simulink model "untitled"  (R2019b)
settings: Solver=VariableStepAuto  StartTime=0.0  StopTime=1.0  RelTol=1e-3
libraries: simulink x1
settings Model: Creator=patti  LastModifiedBy=patti

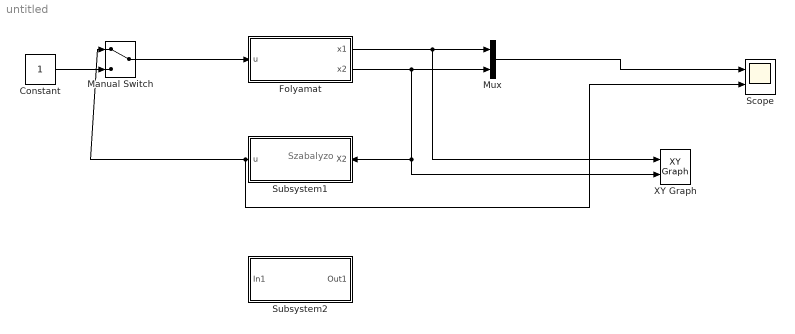
== system untitled ==
  note: Szabalyzo
  Constant : Constant
  "Folyamat " : Subsystem  mask{w=6, x0=[5  ; 8]}
  Manual Switch : ManualSwitch
  Mux : Mux  Inputs=2
  Scope : Scope  NumInputPorts=2
  Subsystem1 : Subsystem
  Subsystem2 : Subsystem
  XY Graph : simulink/Sinks/XY Graph  xmin=-10  xmax=100  ymin=-10  ymax=100  st=0.01
  wires:
  Manual Switch/1 -> "Folyamat "/1(u)
  "Folyamat "/1(x1) -> XY Graph/1, Mux/1
  "Folyamat "/2(x2) -> Mux/2, XY Graph/2, Subsystem1/1(X2)
  Subsystem1/1("u ") -> Scope/2, Manual Switch/1
  Constant/1 -> Manual Switch/2
  Mux/1 -> Scope/1

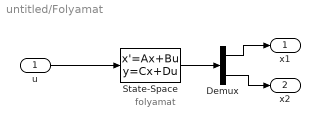
== system untitled/Folyamat  ==
  note: folyamat
  u : Inport
  Demux : Demux  Outputs=2
  State-Space : StateSpace  A=[0 w; -w 0]  B=[0 ; 1]  C=[1 0;0 1]  D=[0 ;0]  InitialCondition=[x0]
  x1 : Outport
  x2 : Outport  Port=2
  wires:
  u/1 -> State-Space/1
  State-Space/1 -> Demux/1
  Demux/1 -> x1/1
  Demux/2 -> x2/1

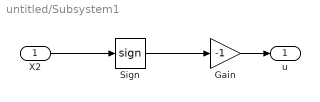
== system untitled/Subsystem1 ==
  X2 : Inport
  Gain : Gain  Gain=-1
  Sign : Signum
  "u " : Outport
  wires:
  X2/1 -> Sign/1
  Sign/1 -> Gain/1
  Gain/1 -> "u "/1

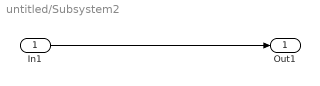
== system untitled/Subsystem2 ==
  In1 : Inport
  Out1 : Outport
  wires:
  In1/1 -> Out1/1
